simulink model "UAV_Taut_Cable"  (R2018a)
settings: Solver=ode4  StartTime=0.0  StopTime=4  FixedStep=1/500  RelTol=1e-3
values from neighbouring files (symbols this model uses):
  alpha_0 = pi/8    (= 0.392699081699)    [UAV_Taut_Cable_parameters.m]
  alpha_bar = 9*pi/10    (= 2.82743338823)    [UAV_Taut_Cable_parameters.m]
  g = 9.81    [UAV_Taut_Cable_parameters.m]
  I = 0.015    [UAV_Taut_Cable_parameters.m]
  k_Da = 2*sqrt(k_Pa)    [UAV_Taut_Cable_parameters.m]
  k_Dr = 2*sqrt(k_Pr)    [UAV_Taut_Cable_parameters.m]
  k_Dt = 2*0.9*sqrt(k_Pr)    [UAV_Taut_Cable_parameters.m]
  k_Pa = 30    [UAV_Taut_Cable_parameters.m]
  k_Pr = 30    [UAV_Taut_Cable_parameters.m]
  k_Pt = 200    [UAV_Taut_Cable_parameters.m]
  m = 2    [UAV_Taut_Cable_parameters.m]
  r_0 = 0.5    [UAV_Taut_Cable_parameters.m]
  r_bar = 0.5    [UAV_Taut_Cable_parameters.m]
  rho = 0.1    [UAV_Taut_Cable_parameters.m]
  T_bar = m*g*(tan(alpha_bar+theta_bar)*cos(alpha_bar) - sin(alpha_bar))    [UAV_Taut_Cable_parameters.m]
  theta_0 = pi/10    (= 0.314159265359)    [UAV_Taut_Cable_parameters.m]
  theta_bar = -pi/20    (= -0.157079632679)    [UAV_Taut_Cable_parameters.m]
undefined symbols (not defined in the file or in its folder): DiscIntNeverNeededParam
libraries: simulink x2
settings Model: Creator=Ahmad  LastModifiedBy=Ahmad

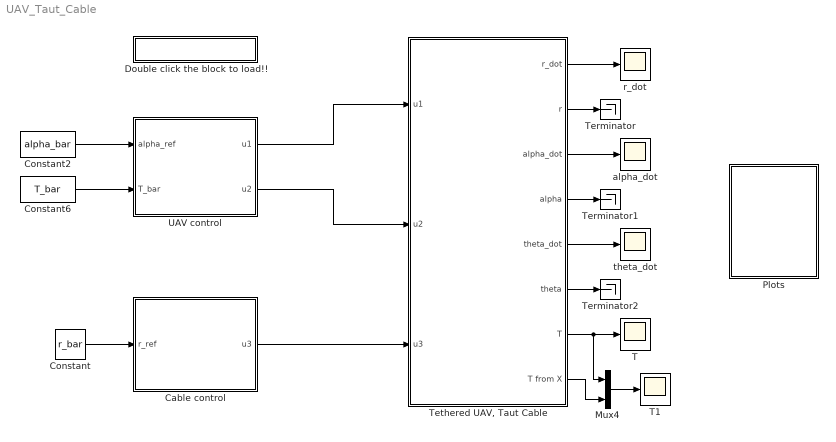
== system UAV_Taut_Cable ==
  Cable control : Subsystem
  Constant : Constant  Value=r_bar
  Constant2 : Constant  Value=alpha_bar
  Constant6 : Constant  Value=T_bar
  Double click the block to load!! : Subsystem
      settings: OpenFcn=UAV_Taut_Cable_parameters
      mask Display:
      | text(.5,.5,'load parameters',...
      | 	'horizontalalignment','center');
  Mux4 : Mux  Inputs=2
  Plots : Subsystem
  T : Scope
  T1 : Scope
  Terminator : Terminator
  Terminator1 : Terminator
  Terminator2 : Terminator
  "Tethered UAV, Taut Cable" : Subsystem
  UAV control : Subsystem
  alpha_dot : Scope
  r_dot : Scope
  theta_dot : Scope
  wires:
  Cable control/1(u3) -> "Tethered UAV, Taut Cable"/3(u3)
  UAV control/1(u1) -> "Tethered UAV, Taut Cable"/1(u1)
  UAV control/2(u2) -> "Tethered UAV, Taut Cable"/2(u2)
  Constant/1 -> Cable control/1(r_ref)
  Constant2/1 -> UAV control/1(alpha_ref)
  Constant6/1 -> UAV control/2(T_bar)
  "Tethered UAV, Taut Cable"/7(T) -> Mux4/1, T/1
  "Tethered UAV, Taut Cable"/5(theta_dot) -> theta_dot/1
  "Tethered UAV, Taut Cable"/3(alpha_dot) -> alpha_dot/1
  "Tethered UAV, Taut Cable"/1(r_dot) -> r_dot/1
  "Tethered UAV, Taut Cable"/8(T from X) -> Mux4/2
  Mux4/1 -> T1/1
  "Tethered UAV, Taut Cable"/2(r) -> Terminator/1
  "Tethered UAV, Taut Cable"/4(alpha) -> Terminator1/1
  "Tethered UAV, Taut Cable"/6(theta) -> Terminator2/1

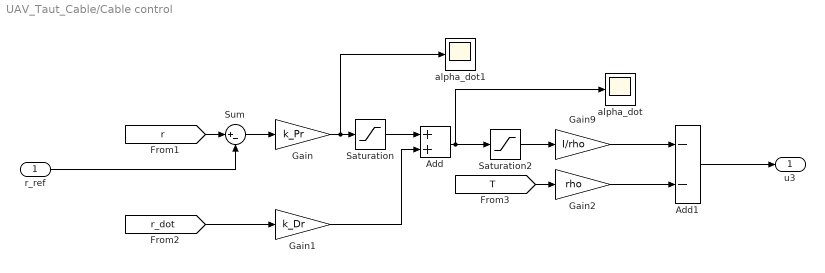
== system UAV_Taut_Cable/Cable control ==
  r_ref : Inport
  Add : Sum
  Add1 : Sum  Inputs=--
  Gain : Gain  Gain=k_Pr
  Gain1 : Gain  Gain=k_Dr
  Gain2 : Gain  Gain=rho
  Gain9 : Gain  Gain=I/rho
  Saturation : Saturate  UpperLimit=15  LowerLimit=-15
  Saturation2 : Saturate  UpperLimit=30  LowerLimit=-30
  Sum : Sum  Inputs=|+-
  alpha_dot : Scope
  alpha_dot1 : Scope
  u3 : Outport
  wires:
  Gain9/1 -> Add1/1
  [r] -> Sum/1
  Saturation/1 -> Add/1
  Gain2/1 -> Add1/2
  Gain1/1 -> Add/2
  [r_dot] -> Gain1/1
  Saturation2/1 -> Gain9/1
  [T] -> Gain2/1
  Sum/1 -> Gain/1
  Gain/1 -> alpha_dot1/1, Saturation/1
  r_ref/1 -> Sum/2
  Add1/1 -> u3/1
  Add/1 -> alpha_dot/1, Saturation2/1

== system UAV_Taut_Cable/Double click the block to load!! ==

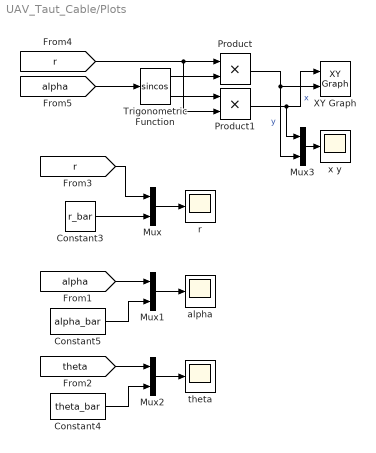
== system UAV_Taut_Cable/Plots ==
  Constant3 : Constant  Value=r_bar
  Constant4 : Constant  Value=theta_bar
  Constant5 : Constant  Value=alpha_bar
  Mux{,1..3} (4 alike) : Mux  Inputs=2
  Product : Product
  Product1 : Product
  Trigonometric Function : Trigonometry  Operator=sincos
  XY Graph : simulink/Sinks/XY Graph  xmin=-1.5  xmax=1.5  ymin=-1.5  ymax=1.5  st=1/50
  alpha : Scope
  r : Scope
  theta : Scope
  x y : Scope
  wires:
  Mux2/1 -> theta/1
  Constant3/1 -> Mux/2
  Mux1/1 -> alpha/1
  [r] -> Product1/2, Product/1
  [alpha] -> Trigonometric Function/1
  Constant5/1 -> Mux1/2
  [alpha] -> Mux1/1
  Trigonometric Function/1 -> Product/2
  [r] -> Mux/1
  Trigonometric Function/2 -> Product1/1
  Product/1 -> Mux3/2, XY Graph/2  "y"
  Mux/1 -> r/1
  Product1/1 -> Mux3/1, XY Graph/1  "x"
  [theta] -> Mux2/1
  Mux3/1 -> x y/1
  Constant4/1 -> Mux2/2

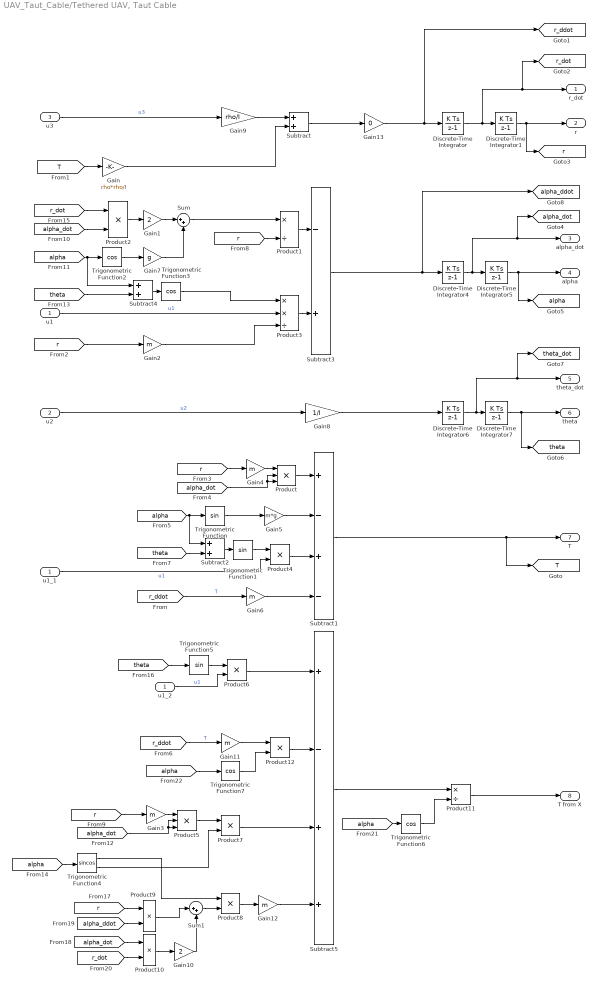
== system UAV_Taut_Cable/Tethered UAV, Taut Cable ==
  u1 : Inport
  u2 : Inport  Port=2
  u3 : Inport  Port=3
  Discrete-Time Integrator : DiscreteIntegrator  SampleTime=-1  ICPrevOutput=DiscIntNeverNeededParam  ICPrevScaledInput=DiscIntNeverNeededParam
  Discrete-Time Integrator1 : DiscreteIntegrator  InitialCondition=r_0  SampleTime=-1  ICPrevOutput=DiscIntNeverNeededParam  ICPrevScaledInput=DiscIntNeverNeededParam
  Discrete-Time Integrator4 : DiscreteIntegrator  SampleTime=-1  ICPrevOutput=DiscIntNeverNeededParam  ICPrevScaledInput=DiscIntNeverNeededParam
  Discrete-Time Integrator5 : DiscreteIntegrator  InitialCondition=alpha_0  SampleTime=-1  ICPrevOutput=DiscIntNeverNeededParam  ICPrevScaledInput=DiscIntNeverNeededParam
  Discrete-Time Integrator6 : DiscreteIntegrator  SampleTime=-1  ICPrevOutput=DiscIntNeverNeededParam  ICPrevScaledInput=DiscIntNeverNeededParam
  Discrete-Time Integrator7 : DiscreteIntegrator  InitialCondition=theta_0  SampleTime=-1  ICPrevOutput=DiscIntNeverNeededParam  ICPrevScaledInput=DiscIntNeverNeededParam
  Gain : Gain  Gain=rho*rho/I
  Gain1 : Gain  Gain=2
  Gain10 : Gain  Gain=2
  Gain{2..4,6,11..12} (6 alike) : Gain  Gain=m
  Gain13 : Gain  Gain=0
  Gain5 : Gain  Gain=m*g
  Gain7 : Gain  Gain=g
  Gain8 : Gain  Gain=1/I
  Gain9 : Gain  Gain=rho/I
  Product : Product  Inputs=3
  Product1 : Product  Inputs=*/
  Product{4,6..10,12} (7 alike) : Product
  Product11 : Product  Inputs=*/
  Product2 : Product  Inputs=**
  Product3 : Product  Inputs=**/
  Product5 : Product  Inputs=3
  Subtract : Sum
  Subtract1 : Sum  Inputs=+-+-
  Subtract2 : Sum
  Subtract3 : Sum  Inputs=-+
  Subtract4 : Sum
  Subtract5 : Sum  Inputs=+-++
  Sum : Sum  Inputs=|++
  Sum1 : Sum  Inputs=|++
  Trigonometric Function : Trigonometry
  Trigonometric Function1 : Trigonometry
  Trigonometric Function{2..3,6..7} (4 alike) : Trigonometry  Operator=cos
  Trigonometric Function4 : Trigonometry  Operator=sincos
  Trigonometric Function5 : Trigonometry
  u1_1 : InportShadow
  u1_2 : InportShadow
  r_dot : Outport
  r : Outport  Port=2
  alpha_dot : Outport  Port=3
  alpha : Outport  Port=4
  theta_dot : Outport  Port=5
  theta : Outport  Port=6
  T : Outport  Port=7
  T from X : Outport  Port=8
  tag scope: T=global, alpha=global, alpha_ddot=global, alpha_dot=global, r=global, r_ddot=global, r_dot=global, theta=global, theta_dot=global
  wires:
  Subtract/1 -> Gain13/1
  Discrete-Time Integrator4/1 -> [alpha_dot], alpha_dot/1, Discrete-Time Integrator5/1
  Discrete-Time Integrator/1 -> [r_dot], r_dot/1, Discrete-Time Integrator1/1
  Product3/1 -> Subtract3/2
  Gain/1 -> Subtract/2
  Subtract4/1 -> Trigonometric Function3/1
  Discrete-Time Integrator1/1 -> r/1, [r]
  Discrete-Time Integrator5/1 -> [alpha], alpha/1
  u3/1 -> Gain9/1  "u3"
  u2/1 -> Gain8/1  "u2"
  Subtract3/1 -> [alpha_ddot], Discrete-Time Integrator4/1
  Trigonometric Function3/1 -> Product3/1
  Discrete-Time Integrator6/1 -> [theta_dot], theta_dot/1, Discrete-Time Integrator7/1
  Discrete-Time Integrator7/1 -> [theta], theta/1
  [alpha] -> Trigonometric Function2/1, Subtract4/1
  [theta] -> Subtract4/2
  Trigonometric Function2/1 -> Gain7/1
  u1/1 -> Product3/2  "u1"
  [T] -> Gain/1
  Gain8/1 -> Discrete-Time Integrator6/1
  Gain9/1 -> Subtract/1
  [r] -> Product1/2
  [r_dot] -> Product2/1
  [alpha_dot] -> Product2/2
  Sum/1 -> Product1/1
  Gain7/1 -> Sum/2
  Product2/1 -> Gain1/1
  Gain1/1 -> Sum/1
  Product1/1 -> Subtract3/1
  [r] -> Gain2/1
  Gain2/1 -> Product3/3
  Trigonometric Function1/1 -> Product4/1
  Gain5/1 -> Subtract1/2
  [alpha_dot] -> Product/2, Product/3
  [alpha] -> Trigonometric Function/1, Subtract2/1
  Subtract2/1 -> Trigonometric Function1/1
  [r] -> Gain4/1
  Subtract1/1 -> [T], T/1
  [theta] -> Subtract2/2
  Gain4/1 -> Product/1
  Product4/1 -> Subtract1/3
  Product/1 -> Subtract1/1
  [r_ddot] -> Gain6/1  "T"
  Trigonometric Function/1 -> Gain5/1
  Gain6/1 -> Subtract1/4
  [r_ddot] -> Gain11/1  "T"
  u1_1/1 -> Product4/2  "u1"
  Gain3/1 -> Product5/1
  Product11/1 -> T from X/1
  [r] -> Gain3/1
  [theta] -> Trigonometric Function5/1
  [alpha] -> Trigonometric Function4/1
  [alpha_dot] -> Product5/3, Product5/2
  Trigonometric Function5/1 -> Product6/1
  Product5/1 -> Product7/1
  Trigonometric Function4/2 -> Product7/2
  Product8/1 -> Gain12/1
  Trigonometric Function4/1 -> Product8/1
  [r] -> Product9/1
  Sum1/1 -> Product8/2
  [alpha_ddot] -> Product9/2
  u1_2/1 -> Product6/2  "u1"
  Product9/1 -> Sum1/1
  [alpha_dot] -> Product10/1
  Product10/1 -> Gain10/1
  Gain10/1 -> Sum1/2
  [r_dot] -> Product10/2
  Subtract5/1 -> Product11/1
  [alpha] -> Trigonometric Function6/1
  Trigonometric Function6/1 -> Product11/2
  Product6/1 -> Subtract5/1
  Product12/1 -> Subtract5/2
  Gain12/1 -> Subtract5/4
  Product7/1 -> Subtract5/3
  [alpha] -> Trigonometric Function7/1
  Gain11/1 -> Product12/1
  Trigonometric Function7/1 -> Product12/2
  Gain13/1 -> [r_ddot], Discrete-Time Integrator/1

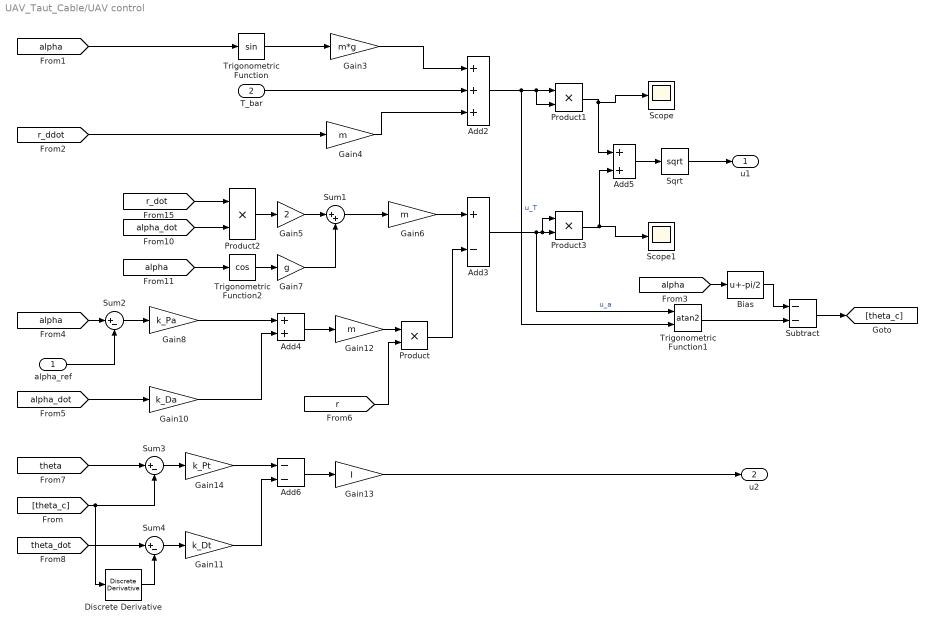
== system UAV_Taut_Cable/UAV control ==
  alpha_ref : Inport
  T_bar : Inport  Port=2
  Add2 : Sum  Inputs=+++
  Add3 : Sum  Inputs=+-
  Add4 : Sum
  Add5 : Sum  Inputs=2
  Add6 : Sum  Inputs=--
  Bias : Bias  Bias=-pi/2
  Discrete Derivative : simulink/Discrete/Discrete Derivative  gainval=1.0  ICPrevScaledInput=0.0  OutMin=[]  OutMax=[]  OutDataType=fixdt(1, 16)  OutScaling=2^-10  DoSatur=off
  Gain10 : Gain  Gain=k_Da
  Gain11 : Gain  Gain=k_Dt
  Gain12 : Gain  Gain=m
  Gain13 : Gain  Gain=I
  Gain14 : Gain  Gain=k_Pt
  Gain3 : Gain  Gain=m*g
  Gain4 : Gain  Gain=m
  Gain5 : Gain  Gain=2
  Gain6 : Gain  Gain=m
  Gain7 : Gain  Gain=g
  Gain8 : Gain  Gain=k_Pa
  Product : Product
  Product1 : Product
  Product2 : Product  Inputs=**
  Product3 : Product
  Scope : Scope
  Scope1 : Scope
  Sqrt : Sqrt  SaturateOnIntegerOverflow=on
  Subtract : Sum  Inputs=--
  Sum1 : Sum  Inputs=|++
  Sum2 : Sum  Inputs=|+-
  Sum3 : Sum  Inputs=|+-
  Sum4 : Sum  Inputs=|+-
  Trigonometric Function : Trigonometry
  Trigonometric Function1 : Trigonometry  Operator=atan2
  Trigonometric Function2 : Trigonometry  Operator=cos
  u1 : Outport
  u2 : Outport  Port=2
  wires:
  [alpha] -> Trigonometric Function/1
  Trigonometric Function/1 -> Gain3/1
  Gain3/1 -> Add2/1
  T_bar/1 -> Add2/2
  [r_ddot] -> Gain4/1
  Gain4/1 -> Add2/3
  Trigonometric Function2/1 -> Gain7/1
  [alpha] -> Trigonometric Function2/1
  Gain5/1 -> Sum1/1
  Gain7/1 -> Sum1/2
  Product2/1 -> Gain5/1
  [alpha_dot] -> Product2/2
  [r_dot] -> Product2/1
  Sum1/1 -> Gain6/1
  Gain6/1 -> Add3/1
  Gain12/1 -> Product/1
  [alpha] -> Sum2/1
  Gain8/1 -> Add4/1
  Gain10/1 -> Add4/2
  [alpha_dot] -> Gain10/1
  Add4/1 -> Gain12/1
  Sum2/1 -> Gain8/1
  alpha_ref/1 -> Sum2/2
  [r] -> Product/2
  Product/1 -> Add3/2
  Add2/1 -> Trigonometric Function1/2, Product1/2, Product1/1  "u_T"
  Add3/1 -> Trigonometric Function1/1, Product3/1, Product3/2  "u_a"
  Product1/1 -> Scope/1, Add5/1
  Product3/1 -> Scope1/1, Add5/2
  Add5/1 -> Sqrt/1
  Sqrt/1 -> u1/1
  [theta_c] -> Discrete Derivative/1, Sum3/2
  Sum3/1 -> Gain14/1
  Add6/1 -> Gain13/1
  [theta_dot] -> Sum4/1
  Gain11/1 -> Add6/2
  Gain14/1 -> Add6/1
  [theta] -> Sum3/1
  Gain13/1 -> u2/1
  Sum4/1 -> Gain11/1
  Discrete Derivative/1 -> Sum4/2
  Trigonometric Function1/1 -> Subtract/2
  [alpha] -> Bias/1
  Bias/1 -> Subtract/1
  Subtract/1 -> [theta_c]
